simulink model "parameters"  (R2021a)
settings: Solver=VariableStepAuto  StartTime=0.0  StopTime=10.0  RelTol=1e-3
model workspace (MAT data in the model file):
  C1_weight = Simulink.Parameter
  C1_weight.Value = 0.5
  C1_weight.DataType = 'auto'
  C1_weight.Dimensions = [1 1]
  controllerBandwidth = Simulink.Parameter
  controllerBandwidth.Value = 0.2
  controllerBandwidth.DataType = 'auto'
  controllerBandwidth.Dimensions = [1 1]
  dampingRatio = Simulink.Parameter
  dampingRatio.Value = 1
  dampingRatio.DataType = 'auto'
  dampingRatio.Dimensions = [1 1]
  precVehicleLenght = Simulink.Parameter
  precVehicleLenght.Value = 4
  precVehicleLenght.DataType = 'auto'
  precVehicleLenght.Dimensions = [1 1]
  targetDistance = Simulink.Parameter
  targetDistance.Value = 15
  targetDistance.DataType = 'auto'
  targetDistance.Dimensions = [1 1]
settings Model: ParameterArgumentNames=C1_weight,controllerBandwidth,dampingRatio,precVehicleLenght,targetDistance  OrderedModelArguments=off  Creator=maurizio  LastModifiedBy=maurizio

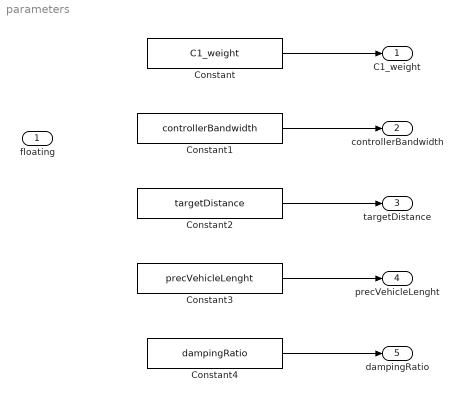
== system parameters ==
  floating : Inport
  Constant : Constant  Value=C1_weight
  Constant1 : Constant  Value=controllerBandwidth
  Constant2 : Constant  Value=targetDistance
  Constant3 : Constant  Value=precVehicleLenght
  Constant4 : Constant  Value=dampingRatio
  C1_weight : Outport
  controllerBandwidth : Outport  Port=2
  targetDistance : Outport  Port=3
  precVehicleLenght : Outport  Port=4
  dampingRatio : Outport  Port=5
  wires:
  Constant/1 -> C1_weight/1
  Constant1/1 -> controllerBandwidth/1
  Constant2/1 -> targetDistance/1
  Constant3/1 -> precVehicleLenght/1
  Constant4/1 -> dampingRatio/1
